simulink model "Q1m"  (R2022a)
settings: Solver=VariableStepAuto  StartTime=0.0  StopTime=10  FixedStep=1e-12  RelTol=1e-6
values from neighbouring files (symbols this model uses):
  C = [1 0 0 0 ... (first row only)    [Q1.m]    (also in Q2.m = [-x4*(2*x3+x4)*sin(x2))
  Kd = dlqr(Ad,Bd,Qd,Rd)    [Q1.m]
  Kdm = dlqr(Adm,Bdm,Qm,Rm)    [Q1.m]
  Kekf = dlqr(Ad,Bd,Qekf,Rekf)    [Q1.m]
  Kkf = dlqr(Ad,Bd,Qkf,Rkf)    [Q1.m]
  Ld = dlqr(Ad',C',V1,V2)'    [Q1.m]
  P0ekf = 1e8*eye(4)    [Q1.m]
  Ts = 5e-3    (= 0.005)    [Q1.m]
  Tsm = 11e-3    (= 0.011)    [Q1.m]
  x0ekf = [deg2rad(0);0;0;0]    [Q1.m]
  x0obs = [deg2rad(0);0;0;0]    [Q1.m]
undefined symbols (not defined in the file or in its folder): Ad, Bd
settings Model: Creator=gusta  LastModifiedBy=gusta

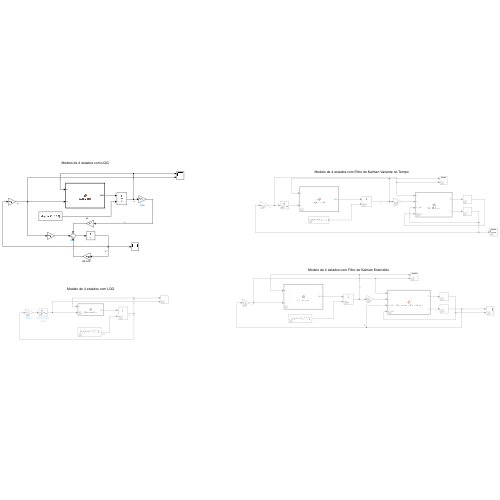
[thumbnail: Simulink's stored preview of the top-level diagram]
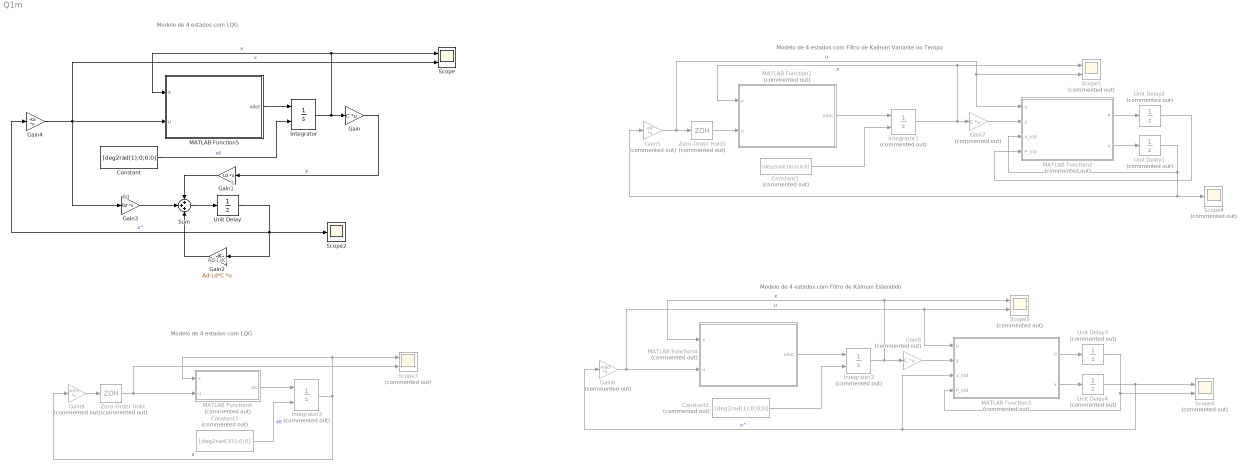
== system Q1m ==
  note: Modelo de 4 estados com LQG
  note: Ad-LdC
  note: Bd
  note: L
  note: Modelo de 4 estados com Filtro de Kalman Variante no Tempo
  note: Modelo de 4 estados com Filtro de Kalman Estendido
  note: Modelo de 4 estados com LQG
  Constant : Constant  Value=[deg2rad(1);0;0;0]
  Constant1 : Constant  Commented=on  Value=[deg2rad(10);0;0;0]
  Constant2 : Constant  Commented=on  Value=[deg2rad(1);0;0;0]
  Constant3 : Constant  Commented=on  Value=[deg2rad(15);0;0]
  Gain : Gain  Gain=C  Multiplication=Matrix(K*u)
  Gain1 : Gain  Gain=Ld  Multiplication=Matrix(K*u)
  Gain2 : Gain  Gain=Ad-Ld*C  Multiplication=Matrix(K*u)
  Gain3 : Gain  Gain=Bd  Multiplication=Matrix(K*u)
  Gain4 : Gain  Gain=-Kd  Multiplication=Matrix(K*u)
  Gain5 : Gain  Commented=on  Gain=-Kkf  Multiplication=Matrix(K*u)
  Gain6 : Gain  Commented=on  Gain=-Kekf  Multiplication=Matrix(K*u)
  Gain7 : Gain  Commented=on  Gain=C  Multiplication=Matrix(K*u)
  Gain8 : Gain  Commented=on  Gain=C  Multiplication=Matrix(K*u)
  Gain9 : Gain  Commented=on  Gain=-Kdm  Multiplication=Matrix(K*u)
  Integrator : Integrator  InitialConditionSource=external
  Integrator1 : Integrator  Commented=on  InitialConditionSource=external
  Integrator2 : Integrator  Commented=on  InitialConditionSource=external
  Integrator3 : Integrator  Commented=on  InitialConditionSource=external
  MATLAB Function1 : MATLAB Function  Commented=on  TreatAsAtomicUnit=on
  MATLAB Function2 : MATLAB Function  Commented=on  TreatAsAtomicUnit=on
  MATLAB Function3 : MATLAB Function  Commented=on  TreatAsAtomicUnit=on
  MATLAB Function4 : MATLAB Function  Commented=on  TreatAsAtomicUnit=on
  MATLAB Function5 : MATLAB Function  TreatAsAtomicUnit=on
  MATLAB Function6 : MATLAB Function  Commented=on  TreatAsAtomicUnit=on
  Scope : Scope  NumInputPorts=2
  Scope{1,3,5..6} (4 alike) : Scope  Commented=on  NumInputPorts=2
  Scope2 : Scope
  Scope4 : Scope  Commented=on
  Sum : Sum  Inputs=+++
  Unit Delay : UnitDelay  InitialCondition=x0obs  SampleTime=-1  HasFrameUpgradeWarning=on
  Unit Delay1 : UnitDelay  Commented=on  InitialCondition=[0;0;0;0]  SampleTime=Ts  HasFrameUpgradeWarning=on
  Unit Delay2 : UnitDelay  Commented=on  SampleTime=Ts  HasFrameUpgradeWarning=on
  Unit Delay3 : UnitDelay  Commented=on  InitialCondition=P0ekf  SampleTime=Ts  HasFrameUpgradeWarning=on
  Unit Delay4 : UnitDelay  Commented=on  InitialCondition=x0ekf  SampleTime=Ts  HasFrameUpgradeWarning=on
  Zero-Order Hold : ZeroOrderHold  Commented=on  SampleTime=Tsm
  Zero-Order Hold1 : ZeroOrderHold  Commented=on  SampleTime=Ts
  wires:
  MATLAB Function5/1(xdot) -> Integrator/1
  Constant/1 -> Integrator/2  "x0"
  Integrator/1 -> Gain/1, Scope/1, MATLAB Function5/1(x)  "x"
  Gain/1 -> Gain1/1  "y"
  Sum/1 -> Unit Delay/1
  Unit Delay/1 -> Gain2/1, Gain4/1, Scope2/1  "x^"
  Gain2/1 -> Sum/3
  Gain3/1 -> Sum/2
  Gain1/1 -> Sum/1
  MATLAB Function2/2(x) -> Unit Delay1/1
  MATLAB Function2/1(P) -> Unit Delay2/1
  Unit Delay2/1 -> MATLAB Function2/4(P_old)
  MATLAB Function1/1(xdot) -> Integrator1/1
  Constant1/1 -> Integrator1/2
  Integrator1/1 -> Gain7/1, MATLAB Function1/1(x), Scope1/1  "x"
  Gain5/1 -> MATLAB Function2/1(u), Scope1/2, Zero-Order Hold1/1  "u"
  Unit Delay1/1 -> Scope4/1, Gain5/1, MATLAB Function2/3(x_old)
  Constant2/1 -> Integrator2/2
  MATLAB Function3/1(P) -> Unit Delay3/1
  MATLAB Function3/2(x) -> Unit Delay4/1
  Gain6/1 -> MATLAB Function4/2(u), MATLAB Function3/1(u), Scope5/2  "u"
  Unit Delay4/1 -> Gain6/1, MATLAB Function3/3(x_old), Scope6/1  "x^"
  Unit Delay3/1 -> Scope6/2, MATLAB Function3/4(P_old)
  Integrator2/1 -> MATLAB Function4/1(x), Scope5/1, Gain8/1  "x"
  Gain7/1 -> MATLAB Function2/2(y)
  Zero-Order Hold1/1 -> MATLAB Function1/2(u)
  Gain8/1 -> MATLAB Function3/2(y)
  MATLAB Function4/1(xdot) -> Integrator2/1
  Gain4/1 -> Gain3/1, Scope/2, MATLAB Function5/2(u)  "u"
  MATLAB Function6/1(dx) -> Integrator3/1
  Constant3/1 -> Integrator3/2  "x0"
  Gain9/1 -> Zero-Order Hold/1
  Integrator3/1 -> Scope3/1, MATLAB Function6/1(x), Gain9/1  "x"
  Zero-Order Hold/1 -> Scope3/2, MATLAB Function6/2(u)

== matlab function Q1m/MATLAB Function1 ==
  data: x input; u input; xdot output
function xdot = GyroModel(x,u)
x1 = x(1); x2 = x(2); x3 = x(3); x4 = x(4);

mV = 0.210;  % Massa do veículo sem giro [kg]
mG = 0.123;  % Massa do giro [kg]
mC = 0;
rG = 0.046;  % Raio do giro [m]
aG = 0.005;  % Espessura giro [m]
aV = 0.088;  % Altura veículo [m]
lV = 0.175;  % Largura veículo [m]
dG = 0.054;  % Distância entre centro de massa do giro e eixo de rotação [m]
dV = 0.025;  % Distância entre centro de massa do veículo e eixo de rotação[m]
omega = 2 * 3657 * 0.10472; % Velocidade de rotação do giro [rad/s]
g = 9.81;    % Gravidade [m/s^2]
d1 = 0.025;
d2 = 0.054;

yL = 0;
zL = 0;
mL = 0;

g = 9.81; % [m/s^2] aceleração da gravidade
IG11 = (mG*(rG^2)/4) + (mG*(dG^2)/12); % IG22 = IG11
IG33 = (mG*(rG^2))/2;
IB11 = (1/12) * mV * (lV^2 + aV^2); % eixo X (roll)

IG22 = IG11;
IL11 = 0;

k1 = IB11 + IL11;
k4 = IG11;     % (IC11 + IG11), IC11 = 0
k5 = IG22;     % (IC22 + IG22), IC22 = 0
k6 = IG33;     % (IC33 + IG33), IC33 = 0

k7 = d1 * mV + d2 * (mC + mG);
k8 = d1^2 * mV + d2^2 * (mC + mG);
k9 = k1 + k8 + (yL^2 + zL^2) * mL;
k10 = k4 - k6;

% Symbolic dynamics
c = cos(x2);

M_u = IG33 * omega * c * u;

% State-space model
xdot = [
    x3;
    x4;
    (k7*g*sin(x1)+2*x3*x4*sin(x2)*cos(x2)*k10-x4*cos(x2)*omega*IG33)/(k9+cos(x2)^2*k4+sin(x2)^2*k6);
    (M_u-x3^2*cos(x2)*sin(x2)*k10-x3*omega*cos(x2)*IG33)/(k5);
];
a = 0;

== matlab function Q1m/MATLAB Function5 ==
  data: x input; u input; xdot output
function xdot = GyroModel(x,u)
x1 = x(1); x2 = x(2); x3 = x(3); x4 = x(4);

mV = 0.210;  % Massa do veículo sem giro [kg]
mG = 0.123;  % Massa do giro [kg]
mC = 0;
rG = 0.046;  % Raio do giro [m]
aG = 0.005;  % Espessura giro [m]
aV = 0.088;  % Altura veículo [m]
lV = 0.175;  % Largura veículo [m]
dG = 0.054;  % Distância entre centro de massa do giro e eixo de rotação [m]
dV = 0.025;  % Distância entre centro de massa do veículo e eixo de rotação[m]
omega = 2 * 3657 * 0.10472; % Velocidade de rotação do giro [rad/s]
g = 9.81;    % Gravidade [m/s^2]
d1 = 0.025;
d2 = 0.054;

yL = 0;
zL = 0;
mL = 0;

g = 9.81; % [m/s^2] aceleração da gravidade
IG11 = (mG*(rG^2)/4) + (mG*(dG^2)/12); % IG22 = IG11
IG33 = (mG*(rG^2))/2;
IB11 = (1/12) * mV * (lV^2 + aV^2); % eixo X (roll)

IG22 = IG11;
IL11 = 0;

k1 = IB11 + IL11;
k4 = IG11;     % (IC11 + IG11), IC11 = 0
k5 = IG22;     % (IC22 + IG22), IC22 = 0
k6 = IG33;     % (IC33 + IG33), IC33 = 0

k7 = d1 * mV + d2 * (mC + mG);
k8 = d1^2 * mV + d2^2 * (mC + mG);
k9 = k1 + k8 + (yL^2 + zL^2) * mL;
k10 = k4 - k6;

% Symbolic dynamics
c = cos(x2);

M_u = IG33 * omega * c * u;

% State-space model
xdot = [
    x3;
    x4;
    (k7*g*sin(x1)+2*x3*x4*sin(x2)*cos(x2)*k10-x4*cos(x2)*omega*IG33)/(k9+cos(x2)^2*k4+sin(x2)^2*k6);
    (M_u-x3^2*cos(x2)*sin(x2)*k10-x3*omega*cos(x2)*IG33)/(k5);
];
a = 0;

== matlab function Q1m/MATLAB Function2 ==
  data: P output; u input; y input; x_old input; P_old input; x output
function [P,x] = FiltroKalman(u,y,x_old,P_old)

I = eye(4);

% Sistema Linearizado Discretizado

Ad = [1.0014         0    0.0069   -0.0011;
   -0.0023    1.0000   -0.0155    0.0069;
    0.6526         0    2.2037   -0.5334;
   -1.4711         0   -7.2210    2.2022];


Bd = [-0.0019;
    0.0155;
   -1.2022;
    7.2187];

C = [1 0 0 0; 0 1 0 0; 0 0 1 0];
  
V1 = 1*diag([10,10,10,5]);
V2 = 1e-6*diag([1,1,1]);

% Measurement update
L = (P_old * C') / (C*P_old*C'+V2);
x = x_old + L * (y - C*x_old);
P = (I-L*C)*P_old;

% Time update
x = Ad * x + Bd * u;
P = Ad * P * Ad' + V1;

end

== matlab function Q1m/MATLAB Function3 ==
  data: P output; u input; y input; x_old input; P_old input; x output
function [P,x] = FiltroKalmanEstendido(u,y,x_old,P_old)

I = eye(4);


C = [1 0 0 0; 0 1 0 0; 0 0 1 0];

V1 = diag([1e-6, 1e-6, 5e-4, 1e-3]);  % um pouco mais de incerteza no modelo
V2 = diag([1e-6, 1e-6, 1e-4]);           % Covariância de medição

% Measurement update
L = (P_old * C') / (C*P_old*C'+V2);
x_corr = x_old + L * (y - C*x_old);
P = (I-L*C)*P_old;

x1 = x_corr(1);
x2 = x_corr(2);
x3 = x_corr(3);
x4 = x_corr(4);

  

Ak =[                                                                          1,                                                                                                                                                                                                                                                                                                             0,                                                                                     0.0050,                                                                                                                 0;
                                                                               0,                                                                                                                                                                                                                                                                                                             1,                                                                                          0,                                                                                                            0.0050;
     (5.8330e-04*cos(x1))/(9.4956e-05*cos(x2)^2 + 1.3013e-04*sin(x2)^2 + 0.0012), (0.0050*(0.0997*x4*sin(x2) - 7.0356e-05*x3*x4*cos(x2)^2 + 7.0356e-05*x3*x4*sin(x2)^2))/(9.4956e-05*cos(x2)^2 + 1.3013e-04*sin(x2)^2 + 0.0012) + (3.5178e-07*cos(x2)*sin(x2)*(0.0997*x4*cos(x2) - 0.1167*sin(x1) + 7.0356e-05*x3*x4*cos(x2)*sin(x2)))/(9.4956e-05*cos(x2)^2 + 1.3013e-04*sin(x2)^2 + 0.0012)^2, 1 - (3.5178e-07*x4*cos(x2)*sin(x2))/(9.4956e-05*cos(x2)^2 + 1.3013e-04*sin(x2)^2 + 0.0012), -(0.0050*(0.0997*cos(x2) + 7.0356e-05*x3*cos(x2)*sin(x2)))/(9.4956e-05*cos(x2)^2 + 1.3013e-04*sin(x2)^2 + 0.0012);
                                                                               0,                                                                                                                                                                                                                          0.0019*x3^2*cos(x2)^2 - 0.0019*x3^2*sin(x2)^2 - 5.2484*u*sin(x2) + 5.2484*x3*sin(x2),                                                 0.0037*x3*cos(x2)*sin(x2) - 5.2484*cos(x2),                                                                                                                 1];
Ts = 5e-3;
  

% Time update
x = x_corr + Ts * [x3;x4;-(0.0997*x4*cos(x2) - 0.1167*sin(x1) + 7.0356e-05*x3*x4*cos(x2)*sin(x2))/(9.4956e-05*cos(x2)^2 + 1.3013e-04*sin(x2)^2 + 0.0012);0.3705*cos(x2)*sin(x2)*x3^2 - 1.0497e+03*cos(x2)*x3 + 1.0497e+03*u*cos(x2)];
P = Ak * P * Ak' + V1;

end

== matlab function Q1m/MATLAB Function4 ==
  data: x input; u input; xdot output
function xdot = GyroModel(x,u)
x1 = x(1); x2 = x(2); x3 = x(3); x4 = x(4);

mV = 0.210;  % Massa do veículo sem giro [kg]
mG = 0.123;  % Massa do giro [kg]
mC = 0;
rG = 0.046;  % Raio do giro [m]
aG = 0.005;  % Espessura giro [m]
aV = 0.088;  % Altura veículo [m]
lV = 0.175;  % Largura veículo [m]
dG = 0.054;  % Distância entre centro de massa do giro e eixo de rotação [m]
dV = 0.025;  % Distância entre centro de massa do veículo e eixo de rotação[m]
omega = 2 * 3657 * 0.10472; % Velocidade de rotação do giro [rad/s]
g = 9.81;    % Gravidade [m/s^2]
d1 = 0.025;
d2 = 0.054;

yL = 0;
zL = 0;
mL = 0;

g = 9.81; % [m/s^2] aceleração da gravidade
IG11 = (mG*(rG^2)/4) + (mG*(dG^2)/12); % IG22 = IG11
IG33 = (mG*(rG^2))/2;
IB11 = (1/12) * mV * (lV^2 + aV^2); % eixo X (roll)

IG22 = IG11;
IL11 = 0;

k1 = IB11 + IL11;
k4 = IG11;     % (IC11 + IG11), IC11 = 0
k5 = IG22;     % (IC22 + IG22), IC22 = 0
k6 = IG33;     % (IC33 + IG33), IC33 = 0

k7 = d1 * mV + d2 * (mC + mG);
k8 = d1^2 * mV + d2^2 * (mC + mG);
k9 = k1 + k8 + (yL^2 + zL^2) * mL;
k10 = k4 - k6;

% Symbolic dynamics
c = cos(x2);

M_u = IG33 * omega * c * u;

% State-space model
xdot = [
    x3;
    x4;
    (k7*g*sin(x1)+2*x3*x4*sin(x2)*cos(x2)*k10-x4*cos(x2)*omega*IG33)/(k9+cos(x2)^2*k4+sin(x2)^2*k6);
    (M_u-x3^2*cos(x2)*sin(x2)*k10-x3*omega*cos(x2)*IG33)/(k5);
];
a = 0;

== matlab function Q1m/MATLAB Function6 ==
  data: x input; u input; dx output
function dx = ModeloMoto(x,u)

x1 = x(1);   % rho
x2 = x(2);   % theta
x3 = x(3);   % rhop

mV = 0.210;  % Massa do veículo sem giro [kg]
mG = 0.123;  % Massa do giro [kg]
rG = 0.046;  % Raio do giro [m]
aG = 0.005;  % Espessura giro [m]
aV = 0.088;  % Altura veículo [m]
lV = 0.175;  % Largura veículo [m]
dG = 0.054;  % Distância entre centro de massa do giro e eixo de rotação [m]
dV = 0.025;  % Distância entre centro de massa do veículo e eixo de rotação[m]
w = 2 * 3657 * 0.10472; % Velocidade de rotação do giro [rad/s]
g = 9.81;    % Gravidade [m/s^2]


IG11 = (mG*rG^2/4) + (mG*aG^2/12);
IG33 = (mG*rG^2/2);
IB11 = mV*(aV^2+lV^2)/12;

dx1 = x3;
dx2 = 0 + u;
dx3 = (mV*dV+mG*dG)*g*sin(x1)/(IB11+mV*dV^2+mG*dG^2+IG11*cos(x2)^2+IG33*sin(x2)^2)+((-2*cos(x2)*sin(x2)*(IG33 - IG11)*x3-w*cos(x2)*IG33))/(IB11 + IG11*(cos(x2)^2)+mV*(dV^2)+mG*(dG^2)+IG33*(sin(x2)^2))*u;

dx = [dx1; dx2; dx3];
end
